simulink model "parameter_handler"  (R2023b)
settings: Solver=FixedStepAuto  StartTime=0.0  StopTime=inf  FixedStep=0.01  RelTol=1e-3
InitFcn:
  | myapp = app3;
StartFcn:
  | blk = 'merge_variable_grain/Biquad Filtering/speed_disp';
  | event = 'PostOutputs';
  | listener = @(app,event) updateGUI(myapp);
  | h = add_exec_event_listener(blk, event, listener);
StopFcn:
  | delete(myapp)
model workspace (MAT data in the model file):
  rng_seed = 0
  sample_dim = 0
undefined symbols (not defined in the file or in its folder): rng_seed_f, sample_dim_f
settings Model: ParameterArgumentNames=rng_seed,sample_dim  Creator=The MathWorks, Inc.  LastModifiedBy=Edp
settings SolverCC: AlgebraicLoopSolver=TrustRegion
settings DataIOCC: SaveOutput=off  SaveTime=off  ReturnWorkspaceOutputs=off
settings DebuggingCC: UnconnectedInputMsg=warning  UnconnectedOutputMsg=warning  UnconnectedLineMsg=warning  ArithmeticOperatorsInVariantConditions=warning
settings ModelReferenceCC: EnableRefExpFcnMdlSchedulingChecks=on
settings SFSimCC: SimUseLocalCustomCode=off  CustomCodeUndefinedFunction=UseInterfaceOnly
settings RTWCC: RTWUseLocalCustomCode=off

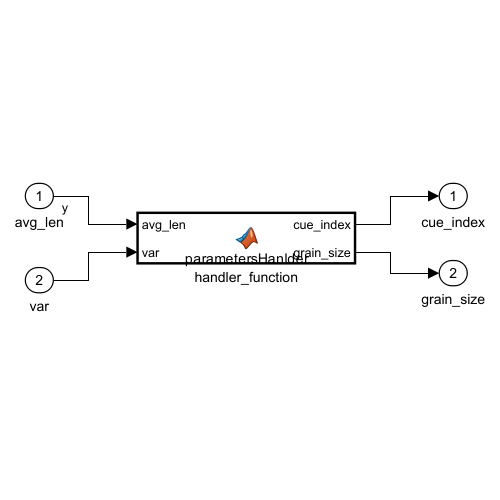
[thumbnail: Simulink's stored preview of the top-level diagram]
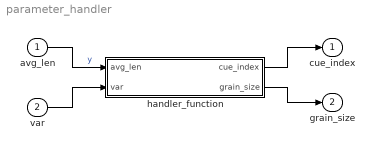
== system parameter_handler ==
  avg_len : Inport  OutDataTypeStr=double  PortDimensions=1  SampleTime=[0.01,0]
  var : Inport  Port=2  OutDataTypeStr=double  PortDimensions=1
  handler_function : MATLAB Function  TreatAsAtomicUnit=on
  cue_index : Outport  OutDataTypeStr=double  PortDimensions=1  SampleTime=[0.01,0]
  grain_size : Outport  Port=2  OutDataTypeStr=double  PortDimensions=1  SampleTime=[0.01,0]
  wires:
  avg_len/1 -> handler_function/1(avg_len)  "y"
  var/1 -> handler_function/2(var)
  handler_function/1(cue_index) -> cue_index/1
  handler_function/2(grain_size) -> grain_size/1

== matlab function parameter_handler/handler_function ==
  data: cue_index output; grain_size output; sample_dim_f parameter; avg_len input; var input; rng_seed_f parameter
% This function takes in input the average length of the grain, adds some
% variation, and outputs the grain size and the cue point of the randomly extracted grain
function [cue_index, grain_size] = parametersHanlder(sample_dim_f, avg_len, var, rng_seed_f)
    rng(rng_seed_f);
    min_grain_size = min(max(avg_len - var, 1), sample_dim_f - 1);
    max_grain_size = max(min(avg_len + var, sample_dim_f - 1), 1);
    cue_index = randi([1, sample_dim_f - floor(max_grain_size)]);
    grain_size = randi([floor(min_grain_size), floor(max_grain_size)]);
end
